simulink model "Debug"  (R2020b)
settings: Solver=VariableStepAuto  StartTime=0.0  StopTime=10.0  RelTol=1e-3
values from neighbouring files (symbols this model uses):
  I_inv = inv(I_mat)    [AngularDynamics_VV.m]
  I_mat = [I_xx I_xy I_xz ... (first row only)    [AngularDynamics_VV.m]    (also in angular_tune_test.m; temp.m)
  M_aerod = [rand*10; rand*10; rand*10]    [AngularDynamics_VV.m]
  pid_Mx = [pid_Mx.Kp, pid_Mx.Ki, pid_Mx.Kd]    [angular_MPC.m]    (also in angular_tune.m)
  pid_My = [pid_My.Kp, pid_My.Ki, pid_My.Kd]    [angular_MPC.m]    (also in angular_tune.m)
  pid_Mz = [pid_Mz.Kp, pid_Mz.Ki, pid_Mz.Kd]    [angular_MPC.m]    (also in angular_tune.m)
  theta_d_0 = [0;0;0]    [AngularDynamics_VV.m]
  theta_desiredV = [rand*pi; rand*pi; rand*pi]    [AngularDynamics_VV.m]
  time_delay = 0.1    [AngularDynamics_VV.m]    (also in LinearDynamics_VV.m = 0)
  w_d_0 = [0;0;0]    [AngularDynamics_VV.m]
libraries: pid_lib x3, sharedutil x1
settings Model: Creator=Jonathan van Zyl  LastModifiedBy=Jonathan van Zyl

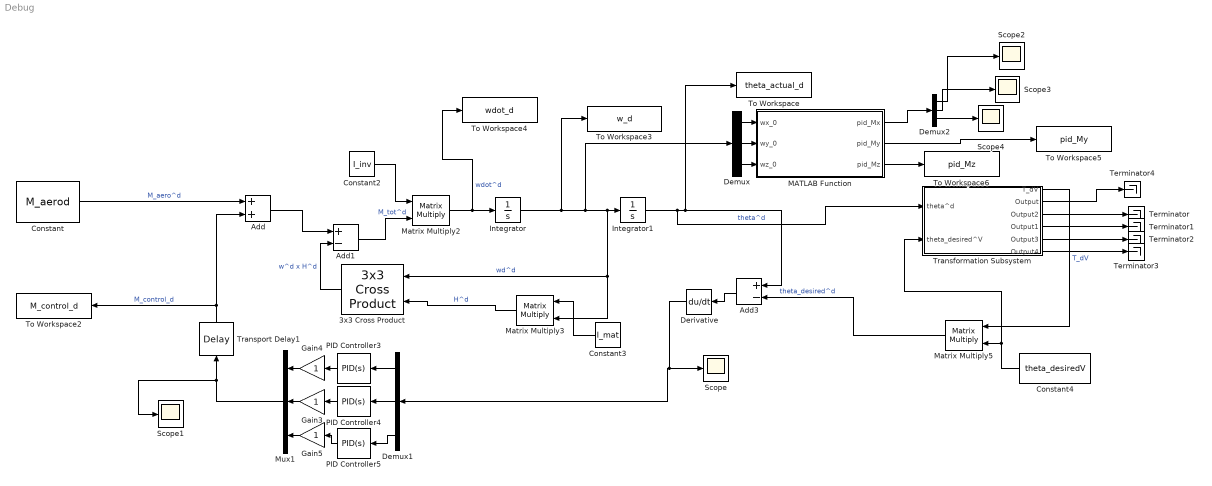
== system Debug ==
  3x3 Cross Product : sharedutil/3x3 Cross Product  aMode=aMode
      settings: SourceProductBaseCode=AE,PW,MT,UV,VE,VP
  Add : Sum
  Add1 : Sum  Inputs=+-
  Add3 : Sum  Inputs=+-
  Constant : Constant  Value=M_aerod
  Constant2 : Constant  Value=I_inv
  Constant3 : Constant  Value=I_mat
  Constant4 : Constant  Value=theta_desiredV
  Demux : Demux  Outputs=3
  Demux1 : Demux  Outputs=3
  Demux2 : Demux  Outputs=3
  Derivative : Derivative
  Gain3 : Gain
  Gain4 : Gain
  Gain5 : Gain
  Integrator : Integrator  InitialCondition=w_d_0
  Integrator1 : Integrator  InitialCondition=theta_d_0
  MATLAB Function : MATLAB Function  TreatAsAtomicUnit=on
  Matrix Multiply2 : Product  Multiplication=Matrix(*)
  Matrix Multiply3 : Product  Multiplication=Matrix(*)
  Matrix Multiply5 : Product  Multiplication=Matrix(*)
  Mux1 : Mux  Inputs=3
  PID Controller3 : pid_lib/PID Controller  Controller=PID  Form=Parallel  TimeDomain=Continuous-time  UseExternalTs=off  SampleTime=-1  IntegratorMethod=Forward Euler  FilterMethod=Forward Euler  ControllerParametersSource=internal  P=pid_Mx(1)  I=pid_Mx(2)  D=pid_Mx(3)  UseFilter=on  N=10.4897155810233  TunerSelectOption=Transfer Function Based (PID Tuner App)  InitialConditionSource=internal  InitialConditionForIntegrator=0  InitialConditionForFilter=0  DifferentiatorICPrevScaledInput=0  ExternalReset=none  TrackingMode=off  Kt=1  LimitOutput=off  SatLimitsSource=internal  UpperSaturationLimit=inf  LowerSaturationLimit=-inf  LinearizeAsGain=on  AntiWindupMode=none  Kb=1  POutMin=[]  POutMax=[]  IOutMin=[]  IOutMax=[]  DOutMin=[]  DOutMax=[]  NOutMin=[]  NOutMax=[]  SumOutMin=[]  SumOutMax=[]  SaturationOutMin=[]  SaturationOutMax=[]  PParamMin=[]  PParamMax=[]  IParamMin=[]  IParamMax=[]  DParamMin=[]  DParamMax=[]  NParamMin=[]  NParamMax=[]  KbParamMin=[]  KbParamMax=[]  KtParamMin=[]  KtParamMax=[]  KbOutMin=[]  KbOutMax=[]  KtOutMin=[]  KtOutMax=[]  IntegratorOutMin=[]  IntegratorOutMax=[]  FilterOutMin=[]  FilterOutMax=[]  SumI1OutMin=[]  SumI1OutMax=[]  SumI2OutMin=[]  SumI2OutMax=[]  SumI3OutMin=[]  SumI3OutMax=[]  SumI4OutMin=[]  SumI4OutMax=[]  SumDOutMin=[]  SumDOutMax=[]  DifferentiatorOutMin=[]  DifferentiatorOutMax=[]  FilterDiffOutCoefMin=[]  FilterDiffOutCoefMax=[]  ReciprocalOutMin=[]  ReciprocalOutMax=[]  SumDenOutMin=[]  SumDenOutMax=[]  SumNumOutMin=[]  SumNumOutMax=[]  DivideOutMin=[]  DivideOutMax=[]  UdiffTsProdOutMin=[]  UdiffTsProdOutMax=[]  NTsProdOutMin=[]  NTsProdOutMax=[]  UintegralTsProdOutMin=[]  UintegralTsProdOutMax=[]  UngainTsProdOutMin=[]  UngainTsProdOutMax=[]  IntegratorContinuousStateAttributes=''  IntegratorStateMustResolveToSignalObject=off  IntegratorRTWStateStorageClass=Auto  FilterContinuousStateAttributes=''  FilterStateMustResolveToSignalObject=off  FilterRTWStateStorageClass=Auto  ParallelPVariant=InternalParameters  IdealPVariant=Disabled  IVariant=InternalParameters  DVariant=InternalParameters  IntegratorVariant=Continuous  SatVariant=Disabled  AWVariant=Passthrough  PCopyVariant=Disabled  TRVariant=Disabled  FdbkBlocksVariant=Forward  IdealPFdbkVariant=Disabled  SatFdbkVariant=Disabled  DerivativeFilterVariant=ContFilter  NVariant=InternalParameters  NCopyVariant=Disabled  FilterICVariant=InternalICsFilter  IntegratorICVariant=InternalICs  ExternalResetVariant=Disabled  TRSumVariant=Passthrough  SumFdbkVariant=Disabled  SumVariant=Sum_PID  TsampFilterVariant=InternalTs  TsampNgainVariant=Passthrough  TsampIntegralVariant=Passthrough  ExternalSaturationOutDataTypeStr=Inherit: Same as second input
  PID Controller4 : pid_lib/PID Controller  Controller=PID  Form=Parallel  TimeDomain=Continuous-time  UseExternalTs=off  SampleTime=-1  IntegratorMethod=Forward Euler  FilterMethod=Forward Euler  ControllerParametersSource=internal  P=pid_My(1)  I=pid_My(2)  D=pid_My(3)  UseFilter=on  N=10.4897155810233  TunerSelectOption=Transfer Function Based (PID Tuner App)  InitialConditionSource=internal  InitialConditionForIntegrator=0  InitialConditionForFilter=0  DifferentiatorICPrevScaledInput=0  ExternalReset=none  TrackingMode=off  Kt=1  LimitOutput=off  SatLimitsSource=internal  UpperSaturationLimit=inf  LowerSaturationLimit=-inf  LinearizeAsGain=on  AntiWindupMode=none  Kb=1  POutMin=[]  POutMax=[]  IOutMin=[]  IOutMax=[]  DOutMin=[]  DOutMax=[]  NOutMin=[]  NOutMax=[]  SumOutMin=[]  SumOutMax=[]  SaturationOutMin=[]  SaturationOutMax=[]  PParamMin=[]  PParamMax=[]  IParamMin=[]  IParamMax=[]  DParamMin=[]  DParamMax=[]  NParamMin=[]  NParamMax=[]  KbParamMin=[]  KbParamMax=[]  KtParamMin=[]  KtParamMax=[]  KbOutMin=[]  KbOutMax=[]  KtOutMin=[]  KtOutMax=[]  IntegratorOutMin=[]  IntegratorOutMax=[]  FilterOutMin=[]  FilterOutMax=[]  SumI1OutMin=[]  SumI1OutMax=[]  SumI2OutMin=[]  SumI2OutMax=[]  SumI3OutMin=[]  SumI3OutMax=[]  SumI4OutMin=[]  SumI4OutMax=[]  SumDOutMin=[]  SumDOutMax=[]  DifferentiatorOutMin=[]  DifferentiatorOutMax=[]  FilterDiffOutCoefMin=[]  FilterDiffOutCoefMax=[]  ReciprocalOutMin=[]  ReciprocalOutMax=[]  SumDenOutMin=[]  SumDenOutMax=[]  SumNumOutMin=[]  SumNumOutMax=[]  DivideOutMin=[]  DivideOutMax=[]  UdiffTsProdOutMin=[]  UdiffTsProdOutMax=[]  NTsProdOutMin=[]  NTsProdOutMax=[]  UintegralTsProdOutMin=[]  UintegralTsProdOutMax=[]  UngainTsProdOutMin=[]  UngainTsProdOutMax=[]  IntegratorContinuousStateAttributes=''  IntegratorStateMustResolveToSignalObject=off  IntegratorRTWStateStorageClass=Auto  FilterContinuousStateAttributes=''  FilterStateMustResolveToSignalObject=off  FilterRTWStateStorageClass=Auto  ParallelPVariant=InternalParameters  IdealPVariant=Disabled  IVariant=InternalParameters  DVariant=InternalParameters  IntegratorVariant=Continuous  SatVariant=Disabled  AWVariant=Passthrough  PCopyVariant=Disabled  TRVariant=Disabled  FdbkBlocksVariant=Forward  IdealPFdbkVariant=Disabled  SatFdbkVariant=Disabled  DerivativeFilterVariant=ContFilter  NVariant=InternalParameters  NCopyVariant=Disabled  FilterICVariant=InternalICsFilter  IntegratorICVariant=InternalICs  ExternalResetVariant=Disabled  TRSumVariant=Passthrough  SumFdbkVariant=Disabled  SumVariant=Sum_PID  TsampFilterVariant=InternalTs  TsampNgainVariant=Passthrough  TsampIntegralVariant=Passthrough  ExternalSaturationOutDataTypeStr=Inherit: Same as second input
  PID Controller5 : pid_lib/PID Controller  Controller=PID  Form=Parallel  TimeDomain=Continuous-time  UseExternalTs=off  SampleTime=-1  IntegratorMethod=Forward Euler  FilterMethod=Forward Euler  ControllerParametersSource=internal  P=pid_Mz(1)  I=pid_Mz(2)  D=pid_Mz(3)  UseFilter=on  N=10.4897155810233  TunerSelectOption=Transfer Function Based (PID Tuner App)  InitialConditionSource=internal  InitialConditionForIntegrator=0  InitialConditionForFilter=0  DifferentiatorICPrevScaledInput=0  ExternalReset=none  TrackingMode=off  Kt=1  LimitOutput=off  SatLimitsSource=internal  UpperSaturationLimit=inf  LowerSaturationLimit=-inf  LinearizeAsGain=on  AntiWindupMode=none  Kb=1  POutMin=[]  POutMax=[]  IOutMin=[]  IOutMax=[]  DOutMin=[]  DOutMax=[]  NOutMin=[]  NOutMax=[]  SumOutMin=[]  SumOutMax=[]  SaturationOutMin=[]  SaturationOutMax=[]  PParamMin=[]  PParamMax=[]  IParamMin=[]  IParamMax=[]  DParamMin=[]  DParamMax=[]  NParamMin=[]  NParamMax=[]  KbParamMin=[]  KbParamMax=[]  KtParamMin=[]  KtParamMax=[]  KbOutMin=[]  KbOutMax=[]  KtOutMin=[]  KtOutMax=[]  IntegratorOutMin=[]  IntegratorOutMax=[]  FilterOutMin=[]  FilterOutMax=[]  SumI1OutMin=[]  SumI1OutMax=[]  SumI2OutMin=[]  SumI2OutMax=[]  SumI3OutMin=[]  SumI3OutMax=[]  SumI4OutMin=[]  SumI4OutMax=[]  SumDOutMin=[]  SumDOutMax=[]  DifferentiatorOutMin=[]  DifferentiatorOutMax=[]  FilterDiffOutCoefMin=[]  FilterDiffOutCoefMax=[]  ReciprocalOutMin=[]  ReciprocalOutMax=[]  SumDenOutMin=[]  SumDenOutMax=[]  SumNumOutMin=[]  SumNumOutMax=[]  DivideOutMin=[]  DivideOutMax=[]  UdiffTsProdOutMin=[]  UdiffTsProdOutMax=[]  NTsProdOutMin=[]  NTsProdOutMax=[]  UintegralTsProdOutMin=[]  UintegralTsProdOutMax=[]  UngainTsProdOutMin=[]  UngainTsProdOutMax=[]  IntegratorContinuousStateAttributes=''  IntegratorStateMustResolveToSignalObject=off  IntegratorRTWStateStorageClass=Auto  FilterContinuousStateAttributes=''  FilterStateMustResolveToSignalObject=off  FilterRTWStateStorageClass=Auto  ParallelPVariant=InternalParameters  IdealPVariant=Disabled  IVariant=InternalParameters  DVariant=InternalParameters  IntegratorVariant=Continuous  SatVariant=Disabled  AWVariant=Passthrough  PCopyVariant=Disabled  TRVariant=Disabled  FdbkBlocksVariant=Forward  IdealPFdbkVariant=Disabled  SatFdbkVariant=Disabled  DerivativeFilterVariant=ContFilter  NVariant=InternalParameters  NCopyVariant=Disabled  FilterICVariant=InternalICsFilter  IntegratorICVariant=InternalICs  ExternalResetVariant=Disabled  TRSumVariant=Passthrough  SumFdbkVariant=Disabled  SumVariant=Sum_PID  TsampFilterVariant=InternalTs  TsampNgainVariant=Passthrough  TsampIntegralVariant=Passthrough  ExternalSaturationOutDataTypeStr=Inherit: Same as second input
  Scope{,1..4} (5 alike) : Scope
  Terminator{,1..4} (5 alike) : Terminator
  To Workspace : ToWorkspace  VariableName=theta_actual_d  SaveFormat=Timeseries  SampleTime=-1
  To Workspace2 : ToWorkspace  VariableName=M_control_d  SaveFormat=Timeseries  SampleTime=-1
  To Workspace3 : ToWorkspace  VariableName=w_d  SaveFormat=Timeseries  SampleTime=-1
  To Workspace4 : ToWorkspace  VariableName=wdot_d  SaveFormat=Timeseries  SampleTime=-1
  To Workspace5 : ToWorkspace  VariableName=pid_My  SampleTime=-1
      settings: Save2DSignal=2-D array (concatenate along first dimension)
  To Workspace6 : ToWorkspace  VariableName=pid_Mz  SampleTime=-1
      settings: Save2DSignal=2-D array (concatenate along first dimension)
  Transformation Subsystem : Subsystem
  Transport Delay1 : TransportDelay  DelayTime=time_delay  TransDelayFeedthrough=on
  wires:
  MATLAB Function/2(pid_My) -> To Workspace5/1
  Demux/1 -> MATLAB Function/1(wx_0)
  Constant/1 -> Add/1  "M_aero^d"
  Constant2/1 -> Matrix Multiply2/1
  PID Controller4/1 -> Gain3/1
  PID Controller5/1 -> Gain5/1
  Demux1/3 -> PID Controller5/1
  Gain5/1 -> Mux1/3
  PID Controller3/1 -> Gain4/1
  Add/1 -> Add1/1
  Transformation Subsystem/4(Output1) -> Terminator1/1
  Matrix Multiply2/1 -> To Workspace4/1, Integrator/1  "wdot^d"
  Transformation Subsystem/3(Output2) -> Terminator/1
  Transformation Subsystem/5(Output3) -> Terminator2/1
  Transport Delay1/1 -> Add/2, To Workspace2/1  "M_control_d"
  Transformation Subsystem/6(Output4) -> Terminator3/1
  MATLAB Function/3(pid_Mz) -> To Workspace6/1
  Demux1/2 -> PID Controller4/1
  Matrix Multiply5/1 -> Add3/2  "theta_desired^d"
  Integrator1/1 -> Transformation Subsystem/1(theta^d), Add3/1, To Workspace/1  "theta^d"
  MATLAB Function/1(pid_Mx) -> Demux2/1
  Add3/1 -> Derivative/1
  3x3 Cross Product/1 -> Add1/2  "w^d x H^d"
  Demux/3 -> MATLAB Function/3(wz_0)
  Demux1/1 -> PID Controller3/1
  Transformation Subsystem/2(Output) -> Terminator4/1
  Add1/1 -> Matrix Multiply2/2  "M_tot^d"
  Mux1/1 -> Scope1/1, Transport Delay1/1
  Gain3/1 -> Mux1/2
  Matrix Multiply3/1 -> 3x3 Cross Product/2  "H^d"
  Transformation Subsystem/1(T_dV) -> Matrix Multiply5/1  "T_dV"
  Integrator/1 -> Demux/1, 3x3 Cross Product/1, Matrix Multiply3/2, Integrator1/1, To Workspace3/1  "wd^d"
  Gain4/1 -> Mux1/1
  Derivative/1 -> Demux1/1, Scope/1
  Demux/2 -> MATLAB Function/2(wy_0)
  Constant4/1 -> Transformation Subsystem/2(theta_desired^V), Matrix Multiply5/2
  Constant3/1 -> Matrix Multiply3/1
  Demux2/1 -> Scope2/1
  Demux2/2 -> Scope3/1
  Demux2/3 -> Scope4/1

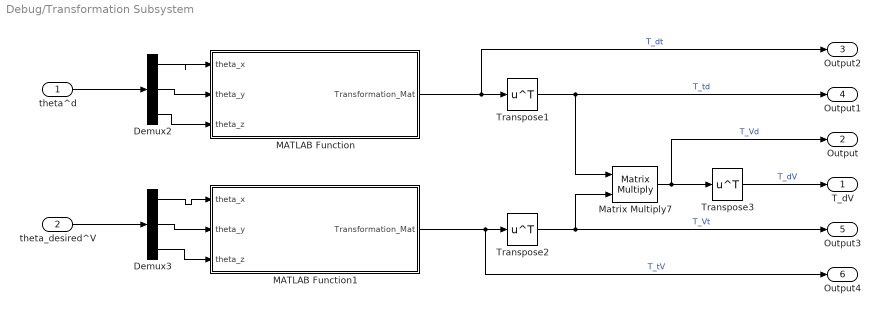
== system Debug/Transformation Subsystem ==
  theta^d : Inport
  theta_desired^V : Inport  Port=2
  Demux2 : Demux  Outputs=3
  Demux3 : Demux  Outputs=3
  MATLAB Function : MATLAB Function  TreatAsAtomicUnit=on
  MATLAB Function1 : MATLAB Function  TreatAsAtomicUnit=on
  Matrix Multiply7 : Product  Multiplication=Matrix(*)
  Transpose1 : Math  Operator=transpose  SaturateOnIntegerOverflow=on
  Transpose2 : Math  Operator=transpose  SaturateOnIntegerOverflow=on
  Transpose3 : Math  Operator=transpose  SaturateOnIntegerOverflow=on
  T_dV : Outport
  Output : Outport  Port=2
  Output2 : Outport  Port=3
  Output1 : Outport  Port=4
  Output3 : Outport  Port=5
  Output4 : Outport  Port=6
  wires:
  Demux3/1 -> MATLAB Function1/1(theta_x)
  Demux2/1 -> MATLAB Function/1(theta_x)
  Transpose2/1 -> Matrix Multiply7/2, Output3/1  "T_Vt"
  Demux2/2 -> MATLAB Function/2(theta_y)
  MATLAB Function/1(Transformation_Mat) -> Output2/1, Transpose1/1  "T_dt"
  Transpose1/1 -> Matrix Multiply7/1, Output1/1  "T_td"
  Demux2/3 -> MATLAB Function/3(theta_z)
  MATLAB Function1/1(Transformation_Mat) -> Output4/1, Transpose2/1  "T_tV"
  Matrix Multiply7/1 -> Output/1, Transpose3/1  "T_Vd"
  theta_desired^V/1 -> Demux3/1
  Demux3/3 -> MATLAB Function1/3(theta_z)
  Demux3/2 -> MATLAB Function1/2(theta_y)
  Transpose3/1 -> T_dV/1  "T_dV"
  theta^d/1 -> Demux2/1

== matlab function Debug/Transformation Subsystem/MATLAB Function ==
  data: theta_x input; Transformation_Mat output; theta_y input; theta_z input
function Transformation_Mat  = Euler(theta_x, theta_y, theta_z)

a = cos(theta_x)*cos(theta_z);
b = cos(theta_x)*sin(theta_z);
c = - sin(theta_x);
d = sin(theta_y)*sin(theta_x)*cos(theta_z) - cos(theta_y)*sin(theta_z);
e = sin(theta_y)*sin(theta_x)*sin(theta_z) + cos(theta_y)*cos(theta_z);
f = sin(theta_y)*cos(theta_x);
g = cos(theta_y)*sin(theta_x)*cos(theta_z) + sin(theta_y)*sin(theta_z);
h = cos(theta_y)*sin(theta_x)*sin(theta_z) - sin(theta_y)*cos(theta_z);
i = cos(theta_y)*cos(theta_x);

Transformation_Mat = [a b c;
    d e f;
    g h i];


end

== matlab function Debug/MATLAB Function ==
  data: wx_0 input; pid_Mx output; wy_0 input; wz_0 input; pid_My output; pid_Mz output
function[pid_Mx, pid_My, pid_Mz] = angular_tune(wx_0, wy_0, wz_0)
%% Load inertias
%Inertia; %A file containing the inertia values, matrix and inverse
global I_xx I_xy I_xz I_yx I_yy I_yz I_zx I_zy I_zz

%% Calculate A matrix
%Calculate numerators
a = (I_yy*I_zz - I_yz*I_zy)*(I_zx*wy_0 - I_yx*wz_0) + (I_xx*I_zy - I_xy*I_zz)*(I_xx*wz_0 - I_zx*wy_0 - I_zz*wz_0) + (I_xy*I_yz - I_xz*I_yy)*(I_zx*wx_0 + I_zy*wy_0 + I_zz*wz_0 - I_yx*wy_0);
b = (I_yy*I_zz - I_yz*I_zy)*(I_zx*wx_0 + I_zy*wy_0 + I_zz*wz_0 - I_yy*wz_0) + (I_xz*I_zy - I_xy*I_zz)*(I_xy*wz_0 - I_zz*wx_0) + (I_xy*I_yz - I_xz*I_yy)*(I_zz*wx_0 - I_yx*wx_0 - I_yy*wy_0 - I_yz*wz_0);
c = (I_yy*I_zz - I_yz*I_zy)*(I_zz*wy_0 - I_yx*wx_0 - I_yy*wy_0 - I_yz*wz_0) + (I_xz*I_zy - I_xy*I_zz)*(I_xx*wx_0 + I_xy*wy_0 + I_xz*wz_0 - I_zz*wx_0) + (I_xy*I_yz - I_xz*I_yy)*(I_zz*wx_0 - I_yz*wy_0);
d = (I_yz*I_zx - I_yx*I_zz)*(I_zx*wy_0 - I_yx*wz_0) + (I_xx*I_zz - I_xz*I_zx)*(I_xx*wz_0 - I_zx*wx_0 - I_zy*wy_0 - I_zz*wz_0) + (I_xz*I_yx - I_xx*I_yz)*(I_zx*wx_0 + I_zz*wz_0 - I_yx*wy_0);
e = (I_yz*I_zx - I_yx*I_zz)*(I_zx*wx_0 + I_zy*wy_0 + I_zz*wz_0 - I_yy*wz_0) + (I_xx*I_zz - I_xz*I_zx)*(I_xy*wz_0 - I_zz*wz_0) + (I_xz*I_yx - I_xx*I_yz)*(I_zz*wx_0 - I_yx*wx_0 - I_yy*wy_0 - I_yz*wz_0);
f = (I_yz*I_zx - I_yx*I_zz)*(I_zz*wy_0 - I_yx*wx_0 - I_yy*wy_0 -I_yz*wz_0) + (I_xx*I_zz - I_xz*I_zx)*(I_xx*wx_0 + I_xy*wy_0 + I_xz*wz_0 - I_zz*wx_0) + (I_xz*I_yx - I_xx*I_yz)*(I_zz*wx_0 - I_yz*wy_0);
g = (I_yx*I_zy - I_yy*I_zx)*(I_zx*wy_0 - I_yx*wz_0) + (I_xy*I_zx - I_xx*I_zy)*(I_xx*wz_0 - I_zx*wx_0 - I_zy*wy_0 - I_zz*wz_0) + (I_xx*I_yy - I_xy*I_yx)*(I_zx*wx_0 + I_zy*wy_0 + I_zz*wz_0 - I_yx*wy_0);
h = (I_yx*I_zy - I_yy*I_zx)*(I_zx*wx_0 + I_zy*wy_0 + I_zz*wz_0 - I_yy*wz_0) + (I_xy*I_zx - I_xx*I_zy)*(I_xy*wz_0 - I_zz*wx_0) + (I_xx*I_yy - I_xy*I_yx)*(I_zz*wx_0 - I_yx*wx_0 - I_yy*wy_0 - I_yz*wz_0);
i = (I_yx*I_zy - I_yy*I_zx)*(I_zz*wy_0 - I_yx*wx_0 - I_yy*wy_0 - I_yz*wz_0) + (I_xy*I_zx - I_xx*I_zy)*(I_xx*wx_0 + I_xy*wy_0 + I_xz*wz_0 - I_zz*wx_0) + (I_xx*I_yy - I_xy*I_yx)*(I_zz*wx_0 - I_yz*wy_0);
%Calculate denominator
A_d= I_xx*I_yy*I_zz + I_xy*I_yz*I_zx + I_xz*I_yx*I_zy - I_zx*I_yy*I_xz - I_zy*I_yz*I_xx - I_zz*I_yx*I_xy;
%Form A-matrix
A_mat = [a/A_d b/A_d c/A_d;
    d/A_d e/A_d f/A_d;
    g h i;];

%% Calculate B-matrix
ab = (I_yy*I_zz - I_yz*I_zy)/A_d;
bb = (I_xz*I_zy - I_xy*I_zz)/A_d;
cb = (I_xy*I_yz - I_xz*I_yy)/A_d;
db = (I_yz*I_zx - I_yx*I_zz)/A_d;
eb = (I_xx*I_zz - I_xz*I_zx)/A_d;
fb = (I_xz*I_yx - I_xx*I_yz)/A_d;
gb = (I_yx*I_zy - I_yy*I_zx)/A_d;
hb = (I_xy*I_zx - I_xx*I_zy)/A_d;
ib = (I_xx*I_yy - I_zy*I_yx)/A_d;

B_mat = [ab bb cb;
    db eb fb;
    gb hb ib;];

%% Make C & D matrix

C = eye(3);
D = zeros(3);

%% Make system

sys = ss(A_mat,B_mat,C,D);
trans_func = tf(sys);

pid_Mx = pidtune(trans_func(1,1), 'PID');
pid_Mx = [pid_Mx.Kp, pid_Mx.Ki, pid_Mx.Kd];

pid_My = pidtune(trans_func(2,2), 'PID');
pid_My = [pid_My.Kp, pid_My.Ki, pid_My.Kd];

pid_Mz = pidtune(trans_func(3,3), 'PID');
pid_Mz = [pid_Mz.Kp, pid_Mz.Ki, pid_Mz.Kd];
end

== matlab function Debug/Transformation Subsystem/MATLAB Function1 ==
  data: theta_x input; Transformation_Mat output; theta_y input; theta_z input
function Transformation_Mat  = Euler(theta_x, theta_y, theta_z)

a = cos(theta_x)*cos(theta_z);
b = cos(theta_x)*sin(theta_z);
c = - sin(theta_x);
d = sin(theta_y)*sin(theta_x)*cos(theta_z) - cos(theta_y)*sin(theta_z);
e = sin(theta_y)*sin(theta_x)*sin(theta_z) + cos(theta_y)*cos(theta_z);
f = sin(theta_y)*cos(theta_x);
g = cos(theta_y)*sin(theta_x)*cos(theta_z) + sin(theta_y)*sin(theta_z);
h = cos(theta_y)*sin(theta_x)*sin(theta_z) - sin(theta_y)*cos(theta_z);
i = cos(theta_y)*cos(theta_x);

Transformation_Mat = [a b c;
    d e f;
    g h i];


end
